simulink model "AmplitudeModulation"  (R2016b)
settings: Solver=VariableStepAuto  StartTime=0.0  StopTime=10.0  RelTol=1e-3
settings Model: Creator=Jawad-PC  LastModifiedBy=Jawad-PC
settings DataIOCC: LimitDataPoints=on  SaveOutput=off  SaveTime=off
settings OptimizationCC: BlockReduction=off  BooleanDataType=off  LifeSpan=inf
settings DebuggingCC: SaveWithParameterizedLinksMsg=none  UnderspecifiedInitializationDetection=Classic  MergeDetectMultiDrivingBlocksExec=none  SignalResolutionControl=TryResolveAllWithWarning  AllowSymbolicDim=off  SFUnexpectedBacktrackingDiag=warning  SFNoUnconditionalDefaultTransitionDiag=warning  SFExecutionAtInitializationDiag=none
settings HardwareCC: TargetUnknown=on
settings GRTTargetCC: TargetLangStandard=C89/C90 (ANSI)  GeneratePreprocessorConditionals=Disable all

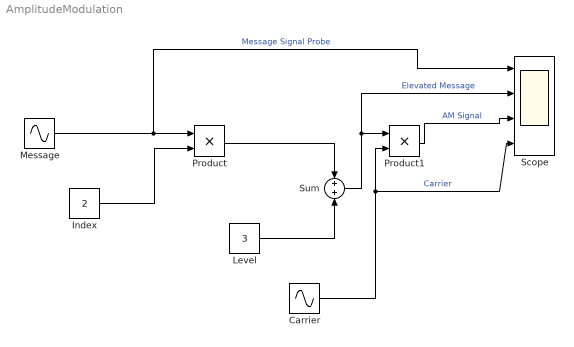
== system AmplitudeModulation ==
  Carrier : Sin  Frequency=20  SampleTime=0
  Index : Constant  Value=2
  Level : Constant  Value=3
  Message : Sin  Frequency=3  SampleTime=0
  Product : Product
  Product1 : Product
  Scope : Scope  NumInputPorts=4
  Sum : Sum  Inputs=2
  wires:
  Message/1 -> Scope/1, Product/1  "Message Signal Probe"
  Index/1 -> Product/2
  Level/1 -> Sum/2
  Product/1 -> Sum/1
  Carrier/1 -> Product1/2, Scope/4  "Carrier"
  Sum/1 -> Product1/1, Scope/2  "Elevated Message"
  Product1/1 -> Scope/3  "AM Signal"
